simulink model "GFOL_nonlinear"  (R2020a)
settings: Solver=ode3  StartTime=0.0  StopTime=Tsim  FixedStep=T_solver  RelTol=1e-6
values from neighbouring files (symbols this model uses):
  f_n1 = f1    (= 50)    [param.m]
  Ipeak_n1 = Sn_n1*sqrt(2)/(sqrt(3)*Un_n1)    [linearization_point.m]    (also in param.m = Sn_n1/(sqrt(3)*Un_n1))
  k_droop_f_n1 = 20*Sn_n1/w_n1    (= 175070.437401)    [param.m]
  k_droop_u_n1 = 0.3*50*Sn_n1/Vpeak_n1    [param.m]
  ki_P_n1 = 1e-3*1/tau_p    (= 0.01)    [param.m]
  ki_pll_n1 = kp_pll_n1/tau_pll_n1    [param.m]
  ki_Q_n1 = 1e-3*1/tau_q    (= 0.01)    [param.m]
  ki_s_n1 = Rc_n1/taus    (= 0.865636363636)    [param.m]
  kp_P_n1 = 1e-3*taus/tau_p    (= 1e-05)    [param.m]
  kp_pll_n1 = xi_pll_n1*2*omega_pll_n1/Vpeak_n1    [param.m]
  kp_Q_n1 = 1e-3*taus/tau_q    (= 1e-05)    [param.m]
  kp_s_n1 = Lc_n1/taus    (= 0.0826621837157)    [param.m]
  Lc_n1 = 0.15*Ln_n1    (= 8.26621837157e-05)    [param.m]
  Lg_n1 = Xg_n1/w_g1    [param.m]
  Lg_n2 = imag(Zg_n2)/w_g1    [param.m]
  P_ref_n1 = 0.5*Sn_n1    (= 1375000)    [param.m]
  plots_step = 10e-6    (= 1e-05)    [param.m]
  Q_ref_n1 = 0.1*Sn_n1    (= 275000)    [param.m]
  Rc_n1 = 0.005*Xn_n1    (= 0.000865636363636)    [param.m]
  Rg_n1 = sqrt(Xcc1^2/(XR_ratio^2+1))    [param.m]
  Rg_n2 = real(Zg_n2)    [param.m]
  Sn_n1 = Sn1    (= 2750000)    [param.m]
  T_solver = 10e-6    (= 1e-05)    [param.m]
  T_step = 2    [param.m]
  tau_droop_f = 1/50    (= 0.02)    [param.m]
  tau_droop_u = 1/50    (= 0.02)    [param.m]
  Vdcref_n1 = 2e3    (= 2000)    [param.m]
  Vpeak_g1_fnl = Vpeak_n1*0.98    [param.m]
  Vpeak_n1 = Un_n1/sqrt(3)*sqrt(2)    [param.m]
  Vpeak_q1_init = Vpeak_n1*1    [param.m]
  w_n1 = 2*pi*f_n1    (= 314.159265359)    [param.m]
undefined symbols (not defined in the file or in its folder): P_set, P_step, Q_set, Q_step, t_ramp, t_step_P, t_step_Q, tau_ramp
libraries: powerlib x37, simulink x5, simulink_extras x1
(part 2 of 2)

== system GFOL_nonlinear/Q loop ==
  Q_ref : Inport
  Q_meas : Inport  Port=2
  u_qd : Inport  Port=3
  is_qd : Inport  Port=4
  Add2 : Sum  Inputs=+-
  Demux2 : Demux  Outputs=2
  Demux7 : Demux  Outputs=2
  Gain12 : Gain  Gain=3/2
  PID Controller : simulink/Continuous/PID Controller  Controller=PI  Form=Parallel  TimeDomain=Continuous-time  UseExternalTs=off  SampleTime=-1  IntegratorMethod=Forward Euler  FilterMethod=Forward Euler  ControllerParametersSource=internal  P=kp_Q_n1  I=ki_Q_n1  D=0  UseFilter=on  N=100  TunerSelectOption=Transfer Function Based (PID Tuner App)  InitialConditionSource=internal  InitialConditionForIntegrator=0  InitialConditionForFilter=0  DifferentiatorICPrevScaledInput=0  ExternalReset=none  TrackingMode=off  Kt=1  LimitOutput=off  UpperSaturationLimit=10*Ipeak_n1  LowerSaturationLimit=-10*Ipeak_n1  LinearizeAsGain=on  AntiWindupMode=clamping  Kb=1  POutMin=[]  POutMax=[]  IOutMin=[]  IOutMax=[]  DOutMin=[]  DOutMax=[]  NOutMin=[]  NOutMax=[]  SumOutMin=[]  SumOutMax=[]  SaturationOutMin=[]  SaturationOutMax=[]  PParamMin=[]  PParamMax=[]  IParamMin=[]  IParamMax=[]  DParamMin=[]  DParamMax=[]  NParamMin=[]  NParamMax=[]  KbParamMin=[]  KbParamMax=[]  KtParamMin=[]  KtParamMax=[]  KbOutMin=[]  KbOutMax=[]  KtOutMin=[]  KtOutMax=[]  IntegratorOutMin=[]  IntegratorOutMax=[]  FilterOutMin=[]  FilterOutMax=[]  SumI1OutMin=[]  SumI1OutMax=[]  SumI2OutMin=[]  SumI2OutMax=[]  SumI3OutMin=[]  SumI3OutMax=[]  SumI4OutMin=[]  SumI4OutMax=[]  SumDOutMin=[]  SumDOutMax=[]  DifferentiatorOutMin=[]  DifferentiatorOutMax=[]  FilterDiffOutCoefMin=[]  FilterDiffOutCoefMax=[]  ReciprocalOutMin=[]  ReciprocalOutMax=[]  SumDenOutMin=[]  SumDenOutMax=[]  SumNumOutMin=[]  SumNumOutMax=[]  DivideOutMin=[]  DivideOutMax=[]  UdiffTsProdOutMin=[]  UdiffTsProdOutMax=[]  NTsProdOutMin=[]  NTsProdOutMax=[]  UintegralTsProdOutMin=[]  UintegralTsProdOutMax=[]  UngainTsProdOutMin=[]  UngainTsProdOutMax=[]  IntegratorContinuousStateAttributes=''  IntegratorStateMustResolveToSignalObject=off  IntegratorRTWStateStorageClass=Auto  FilterContinuousStateAttributes=''  FilterStateMustResolveToSignalObject=off  FilterRTWStateStorageClass=Auto  ParallelPVariant=InternalParameters  IdealPVariant=Disabled  IVariant=InternalParameters  DVariant=Disabled  IntegratorVariant=Continuous  SatVariant=Disabled  AWVariant=Passthrough  PCopyVariant=Disabled  TRVariant=Disabled  FdbkBlocksVariant=Forward  IdealPFdbkVariant=Disabled  SatFdbkVariant=Disabled  DerivativeFilterVariant=Disabled  NVariant=Disabled  NCopyVariant=Disabled_SignalSpec  FilterICVariant=Disabled  IntegratorICVariant=InternalICs  ExternalResetVariant=Disabled  TRSumVariant=Passthrough  SumFdbkVariant=Disabled  SumVariant=Sum_PI  TsampFilterVariant=InternalTs  TsampNgainVariant=Passthrough  TsampIntegralVariant=Passthrough
  Product : Product
  Product1 : Product
  Scope3 : Scope
  Sum1 : Sum  Inputs=|+-
  is_d_ref : Outport
  Q : Outport  Port=2
  wires:
  is_qd/1 -> Demux2/1
  u_qd/1 -> Demux7/1
  Add2/1 -> Gain12/1
  Demux7/1 -> Product/1
  Demux2/1 -> Product1/2
  Product/1 -> Add2/1
  Demux2/2 -> Product/2
  Demux7/2 -> Product1/1
  Product1/1 -> Add2/2
  PID Controller/1 -> is_d_ref/1
  Sum1/1 -> Scope3/1, PID Controller/1
  Q_meas/1 -> Q/1, Sum1/2
  Q_ref/1 -> Sum1/1

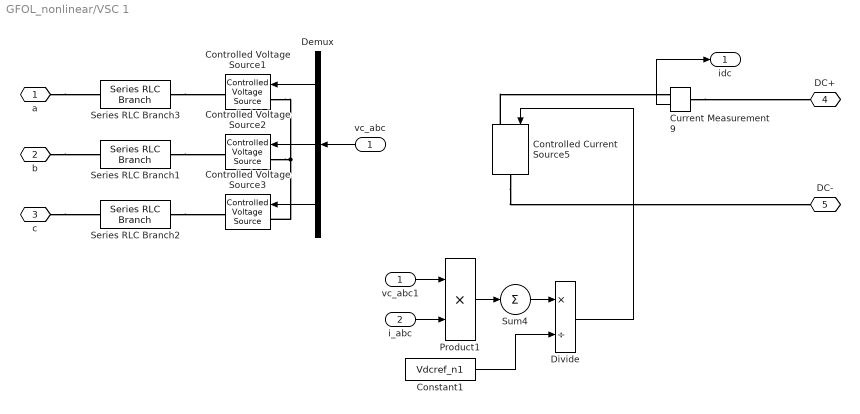
== system GFOL_nonlinear/VSC 1 ==
  vc_abc : Inport
  i_abc : Inport  Port=2
  Constant1 : Constant  Value=Vdcref_n1
  Controlled Current Source5 : powerlib/Electrical Sources/Controlled Current Source  Initialize=on  Source_Type=DC  Amplitude=0  Phase=0  Frequency=0  Measurements=None
  Controlled Voltage Source1 : powerlib/Electrical Sources/Controlled Voltage Source  Initialize=off  Source_Type=AC  Amplitude=0  Phase=0  Frequency=0  Measurements=None
  Controlled Voltage Source2 : powerlib/Electrical Sources/Controlled Voltage Source  Initialize=off  Source_Type=AC  Amplitude=0  Phase=0  Frequency=0  Measurements=None
  Controlled Voltage Source3 : powerlib/Electrical Sources/Controlled Voltage Source  Initialize=off  Source_Type=AC  Amplitude=0  Phase=0  Frequency=0  Measurements=None
  Current Measurement9 : powerlib/Measurements/Current Measurement  PhasorSimulation=off  OutputType=Complex  PSBequivalent=0
  Demux : Demux  Outputs=3
  Divide : Product  Inputs=*/
  Product1 : Product  InputSameDT=on  SaturateOnIntegerOverflow=on  OutDataTypeStr=Inherit: Same as first input
  Series RLC Branch1 : powerlib/Elements/Series RLC Branch  LConnTagsString=__new0  RConnTagsString=__new0  BranchType=R  Resistance=5e-4  Inductance=Lc_n1  SetiL0=off  InitialCurrent=0  Capacitance=0  Setx0=off  InitialVoltage=0  Measurements=None
  Series RLC Branch2 : powerlib/Elements/Series RLC Branch  LConnTagsString=__new0  RConnTagsString=__new0  BranchType=R  Resistance=5e-4  Inductance=Lc_n1  SetiL0=off  InitialCurrent=0  Capacitance=0  Setx0=off  InitialVoltage=0  Measurements=None
  Series RLC Branch3 : powerlib/Elements/Series RLC Branch  LConnTagsString=__new0  RConnTagsString=__new0  BranchType=R  Resistance=5e-4  Inductance=Lc_n1  SetiL0=off  InitialCurrent=0  Capacitance=0  Setx0=off  InitialVoltage=0  Measurements=None
  Sum4 : Sum  Inputs=1  InputSameDT=on  SaturateOnIntegerOverflow=on  OutDataTypeStr=Inherit: Same as first input
  vc_abc1 : InportShadow
  a : PMIOPort  Side=Left
  b : PMIOPort  Port=2  Side=Left
  c : PMIOPort  Port=3  Side=Left
  DC+ : PMIOPort  Port=4  Side=Right
  DC- : PMIOPort  Port=5  Side=Right
  idc : Outport
  wires:
  Current Measurement9/1 -> idc/1
  Product1/1 -> Sum4/1
  Sum4/1 -> Divide/1
  Divide/1 -> Controlled Current Source5/1
  vc_abc1/1 -> Product1/1
  i_abc/1 -> Product1/2
  Demux/2 -> Controlled Voltage Source2/1
  Demux/1 -> Controlled Voltage Source1/1
  Demux/3 -> Controlled Voltage Source3/1
  vc_abc/1 -> Demux/1
  Constant1/1 -> Divide/2
  connections:
  Controlled Current Source5/RConn1 -- DC-/RConn1
  Controlled Current Source5/LConn1 -- Current Measurement9/RConn1
  Current Measurement9/LConn1 -- DC+/RConn1
  a/RConn1 -- Series RLC Branch3/LConn1
  b/RConn1 -- Series RLC Branch1/LConn1
  c/RConn1 -- Series RLC Branch2/LConn1
  Controlled Voltage Source1/LConn1 -- Controlled Voltage Source2/LConn1 -- Controlled Voltage Source3/LConn1
  Series RLC Branch3/RConn1 -- Controlled Voltage Source1/RConn1
  Series RLC Branch1/RConn1 -- Controlled Voltage Source2/RConn1
  Series RLC Branch2/RConn1 -- Controlled Voltage Source3/RConn1

== system GFOL_nonlinear/Current loop/ParkInverse ==
  ABC vector : Inport
  angle : Inport  Port=2
  Constant4 : Constant  Value=2*pi/3
  Constant5 : Constant  Value=2*pi/3
  Constant9 : Constant
  Matrix Concatenate2 : Concatenate  NumInputs=3  Mode=Multidimensional array  ConcatenateDimension=2
  Mux6 : Mux  Inputs=3
  Mux7 : Mux  Inputs=3
  Product : Product  Multiplication=Matrix(*)  RndMeth=Zero
  Sum : Sum  Inputs=|+-
  Sum1 : Sum  Inputs=|++
  Trigonometric Function8 : Trigonometry  Operator=cos
  Trigonometric Function9 : Trigonometry
  Matrix : Outport
  wires:
  angle/1 -> Sum1/1, Sum/1, Mux6/1
  Constant5/1 -> Sum1/2
  Constant4/1 -> Sum/2
  Product/1 -> Matrix/1
  ABC vector/1 -> Product/2
  Sum/1 -> Mux6/2
  Sum1/1 -> Mux6/3
  Constant9/1 -> Mux7/3, Mux7/1, Mux7/2
  Trigonometric Function8/1 -> Matrix Concatenate2/1
  Trigonometric Function9/1 -> Matrix Concatenate2/2
  Mux6/1 -> Trigonometric Function9/1, Trigonometric Function8/1
  Mux7/1 -> Matrix Concatenate2/3
  Matrix Concatenate2/1 -> Product/1

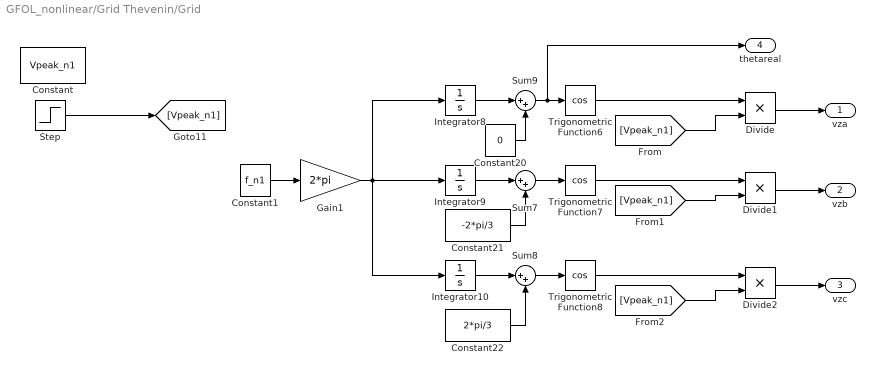
== system GFOL_nonlinear/Grid Thevenin/Grid ==
  Constant : Constant  Value=Vpeak_n1
  Constant1 : Constant  Value=f_n1
  Constant20 : Constant  Value=0
  Constant21 : Constant  Value=-2*pi/3
  Constant22 : Constant  Value=2*pi/3
  Divide : Product  Inputs=**
  Divide1 : Product  Inputs=**
  Divide2 : Product  Inputs=**
  Gain1 : Gain  Gain=2*pi
  Integrator10 : Integrator
  Integrator8 : Integrator
  Integrator9 : Integrator
  Step : Step  Time=T_step  Before=Vpeak_q1_init  After=Vpeak_g1_fnl  SampleTime=0
  Sum7 : Sum  Inputs=|++
  Sum8 : Sum  Inputs=|++
  Sum9 : Sum  Inputs=|++
  Trigonometric Function6 : Trigonometry  Operator=cos
  Trigonometric Function7 : Trigonometry  Operator=cos
  Trigonometric Function8 : Trigonometry  Operator=cos
  vza : Outport
  vzb : Outport  Port=2
  vzc : Outport  Port=3
  thetareal : Outport  Port=4
  wires:
  Constant1/1 -> Gain1/1
  Sum9/1 -> thetareal/1, Trigonometric Function6/1
  Constant22/1 -> Sum8/2
  Integrator10/1 -> Sum8/1
  Constant21/1 -> Sum7/2
  Integrator8/1 -> Sum9/1
  Gain1/1 -> Integrator8/1, Integrator9/1, Integrator10/1
  Sum7/1 -> Trigonometric Function7/1
  Constant20/1 -> Sum9/2
  Integrator9/1 -> Sum7/1
  Sum8/1 -> Trigonometric Function8/1
  Trigonometric Function6/1 -> Divide/1
  Trigonometric Function7/1 -> Divide1/1
  Trigonometric Function8/1 -> Divide2/1
  Step/1 -> [Vpeak_n1]
  Divide/1 -> vza/1
  Divide1/1 -> vzb/1
  Divide2/1 -> vzc/1
  [Vpeak_n1] -> Divide/2
  [Vpeak_n1] -> Divide1/2
  [Vpeak_n1] -> Divide2/2

== system GFOL_nonlinear/PLL/ParkTransform ==
  ABC vector : Inport
  angle : Inport  Port=2
  Constant1 : Constant  Value=1/2
  Constant2 : Constant  Value=1/2
  Constant3 : Constant  Value=2*pi/3
  Constant4 : Constant  Value=2*pi/3
  Constant5 : Constant  Value=1/2
  Gain : Gain  Gain=2/3
  Matrix Concatenate : Concatenate  NumInputs=3  Mode=Multidimensional array  ConcatenateDimension=2
  Mux1 : Mux  Inputs=3
  Mux2 : Mux  Inputs=3
  Mux3 : Mux  Inputs=3
  Product : Product  Multiplication=Matrix(*)  RndMeth=Zero
  Sum : Sum  Inputs=|+-
  Sum1 : Sum  Inputs=|++
  Trigonometric Function1 : Trigonometry  Operator=cos
  Trigonometric Function2 : Trigonometry  Operator=cos
  Trigonometric Function3 : Trigonometry
  Trigonometric Function4 : Trigonometry
  Trigonometric Function5 : Trigonometry  Operator=cos
  Trigonometric Function6 : Trigonometry
  Matrix : Outport
  wires:
  Matrix Concatenate/1 -> Gain/1
  ABC vector/1 -> Product/2
  Product/1 -> Matrix/1
  Gain/1 -> Product/1
  Constant4/1 -> Sum/2
  Constant3/1 -> Sum1/2
  angle/1 -> Trigonometric Function4/1, Trigonometric Function1/1, Sum1/1, Sum/1
  Trigonometric Function3/1 -> Mux1/2
  Trigonometric Function2/1 -> Mux1/1
  Constant2/1 -> Mux1/3
  Sum/1 -> Trigonometric Function3/1, Trigonometric Function2/1
  Trigonometric Function4/1 -> Mux2/2
  Trigonometric Function1/1 -> Mux2/1
  Constant1/1 -> Mux2/3
  Trigonometric Function6/1 -> Mux3/2
  Trigonometric Function5/1 -> Mux3/1
  Constant5/1 -> Mux3/3
  Sum1/1 -> Trigonometric Function6/1, Trigonometric Function5/1
  Mux1/1 -> Matrix Concatenate/2
  Mux2/1 -> Matrix Concatenate/1
  Mux3/1 -> Matrix Concatenate/3
